simulink model "Scenario_TJunction_TrafficLights"  (R2021a)
settings: Solver=VariableStepAuto  StartTime=0.0  StopTime=15  RelTol=1e-3
model workspace (MAT data in the model file):
  Kz_dif = Simulink.Parameter
  Kz_dif.Value = Simulink.data.Expression
  Kz_dif.Value.ExpressionString = " L_dif / (Lc + ds)"
  Kz_dif.DataType = 'auto'
  Kz_dif.Dimensions = -1
  Kz_il = Simulink.Parameter
  Kz_il.Value = Simulink.data.Expression
  Kz_il.Value.ExpressionString = " L_il / (Lc + ds)"
  Kz_il.DataType = 'auto'
  Kz_il.Dimensions = -1
  Kz_ir = Simulink.Parameter
  Kz_ir.Value = Simulink.data.Expression
  Kz_ir.Value.ExpressionString = " L_ir / (Lc + ds)"
  Kz_ir.DataType = 'auto'
  Kz_ir.Dimensions = -1
  Kz_is = Simulink.Parameter
  Kz_is.Value = Simulink.data.Expression
  Kz_is.Value.ExpressionString = " L_is / (Lc + ds)"
  Kz_is.DataType = 'auto'
  Kz_is.Dimensions = -1
  Kz_long = Simulink.Parameter
  Kz_long.Value = Simulink.data.Expression
  Kz_long.Value.ExpressionString = " L_long / (Lc + ds)"
  Kz_long.Description = 'Segmentkapazität (wie viele autos passen hinein)'
  Kz_long.DataType = 'auto'
  Kz_long.Dimensions = -1
  Kz_pre = Simulink.Parameter
  Kz_pre.Value = Simulink.data.Expression
  Kz_pre.Value.ExpressionString = " L_pre / (Lc + ds)"
  Kz_pre.DataType = 'auto'
  Kz_pre.Dimensions = -1
  L_dif = Simulink.Parameter
  L_dif.Value = Simulink.data.Expression
  L_dif.Value.ExpressionString = "L_long-L_pre"
  L_dif.Description = 'Differenz zwischen Abbiegerspurlänge und normaler straßenlänge'
  L_dif.DataType = 'auto'
  L_dif.Dimensions = -1
  L_il = Simulink.Parameter
  L_il.Value = 30
  L_il.Description = 'Länge der innenkreuzungssegments, das linksabbieger durchqueren'
  L_il.DataType = 'auto'
  L_il.Dimensions = [1 1]
  L_ir = Simulink.Parameter
  L_ir.Value = 23
  L_ir.Description = 'Länge der innenkreuzungssegments, das rechtsabbieger durchqueren'
  L_ir.DataType = 'auto'
  L_ir.Dimensions = [1 1]
  L_is = Simulink.Parameter
  L_is.Value = 35
  L_is.Description = 'Länge der innenkreuzungssegments, das geradeausfahrer durchqueren'
  L_is.DataType = 'auto'
  L_is.Dimensions = [1 1]
  L_long = Simulink.Parameter
  L_long.Value = 52.8
  L_long.Description = 'Langes straßensegment  (52.8 meter)'
  L_long.DataType = 'auto'
  L_long.Dimensions = [1 1]
  L_pre = Simulink.Parameter
  L_pre.Value = 20
  L_pre.Description = 'Länge der Abbiegespuren'
  L_pre.DataType = 'auto'
  L_pre.Dimensions = [1 1]
  Lc = Simulink.Parameter
  Lc.Value = 4.4
  Lc.Description = 'Länge eines autos'
  Lc.DataType = 'auto'
  Lc.Dimensions = [1 1]
  Rk = Simulink.Parameter
  Rk.Value = Simulink.data.Expression
  Rk.Value.ExpressionString = " 1 / (Lc / v)"
  Rk.Description = 'Flussrate zwischen den Kanten (bei speed v)'
  Rk.DataType = 'auto'
  Rk.Dimensions = -1
  Tz_dif = Simulink.Parameter
  Tz_dif.Value = Simulink.data.Expression
  Tz_dif.Value.ExpressionString = " L_dif / v"
  Tz_dif.DataType = 'auto'
  Tz_dif.Dimensions = -1
  Tz_il = Simulink.Parameter
  Tz_il.Value = Simulink.data.Expression
  Tz_il.Value.ExpressionString = " L_il / v"
  Tz_il.DataType = 'auto'
  Tz_il.Dimensions = -1
  Tz_ir = Simulink.Parameter
  Tz_ir.Value = Simulink.data.Expression
  Tz_ir.Value.ExpressionString = " L_ir / v"
  Tz_ir.DataType = 'auto'
  Tz_ir.Dimensions = -1
  Tz_is = Simulink.Parameter
  Tz_is.Value = Simulink.data.Expression
  Tz_is.Value.ExpressionString = " L_is / v"
  Tz_is.DataType = 'auto'
  Tz_is.Dimensions = -1
  Tz_long = Simulink.Parameter
  Tz_long.Value = Simulink.data.Expression
  Tz_long.Value.ExpressionString = " L_long / v"
  Tz_long.Description = 'Segment durchfahrtzeit: wie lange würde ein auto brauchen,um
    | ungehindert durch das segment zu fahren.'
  Tz_long.DataType = 'auto'
  Tz_long.Dimensions = -1
  Tz_pre = Simulink.Parameter
  Tz_pre.Value = Simulink.data.Expression
  Tz_pre.Value.ExpressionString = " L_pre / v"
  Tz_pre.DataType = 'auto'
  Tz_pre.Dimensions = -1
  ds = Simulink.Parameter
  ds.Value = Simulink.data.Expression
  ds.Value.ExpressionString = "v*dt"
  ds.DataType = 'auto'
  ds.Dimensions = -1
  dt = Simulink.Parameter
  dt.Value = 1
  dt.Description = 'temporaler sicherheitsabstand'
  dt.DataType = 'auto'
  dt.Dimensions = [1 1]
  v = Simulink.Parameter
  v.Value = 13.89
  v.Description = 'geschwindigkeit eines autos
    | (km/h : 3.75 = m/s)
    | 	30km/h = 8,34m/s
    | 	20km/h = 5.56m/s
    | 	50km/h = 13.89m/s
    | '
  v.DataType = 'auto'
  v.Dimensions = [1 1]
libraries: StreetLanesLibrary x36, EdgesLibrary x36, SourcesAndSinksLibrary x12, LightsLibrary x2
settings Model: OrderedModelArguments=off  Creator=phill  LastModifiedBy=mariekutscher
settings SolverCC: ZeroCrossAlgorithm=Adaptive

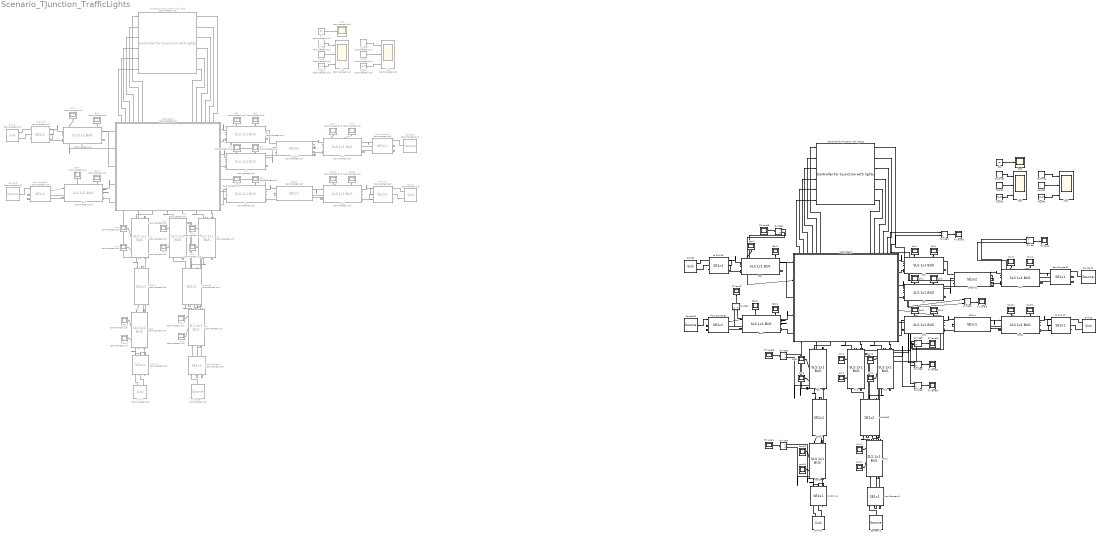
== system Scenario_TJunction_TrafficLights ==
  Ain : StreetLanesLibrary/SLS 1x1 BUS  Commented=on  Kz=Kz_dif  Tz=Tz_dif
  Ain1 : StreetLanesLibrary/SLS 1x1 BUS  Kz=Kz_dif  Tz=Tz_dif
  AinSplit1 : EdgesLibrary/SE1x2  Commented=on  Rk1=0.5*Rk  Rk2=0.5*Rk
  AinSplit2 : EdgesLibrary/SE1x2  Rk1=0.5*Rk  Rk2=0.5*Rk
  AinX : Scope  Commented=on
  AinX1 : Scope
  AinY : Scope  Commented=on
  AinY1 : Scope
  Ali : StreetLanesLibrary/SLS 1x1 BUS  Commented=on  Kz=Kz_pre  Tz=Tz_pre
  Ali1 : StreetLanesLibrary/SLS 1x1 BUS  Kz=Kz_pre  Tz=Tz_pre
  AliX : Scope  Commented=on
  AliX1 : Scope
  AliY : Scope  Commented=on
  AliY1 : Scope
  Ao : StreetLanesLibrary/SLS 1x1 BUS  Commented=on  Kz=Kz_pre  Tz=Tz_pre
  Ao1 : StreetLanesLibrary/SLS 1x1 BUS  Kz=Kz_pre  Tz=Tz_pre
  AoX : Scope  Commented=on
  AoX1 : Scope
  AoY : Scope  Commented=on
  AoY1 : Scope
  Aout : StreetLanesLibrary/SLS 1x1 BUS  Commented=on  Kz=Kz_dif  Tz=Tz_dif
  Aout1 : StreetLanesLibrary/SLS 1x1 BUS  Kz=Kz_dif  Tz=Tz_dif
  AoutX : Scope  Commented=on
  AoutX1 : Scope
  AoutY : Scope  Commented=on
  AoutY1 : Scope
  Ari : StreetLanesLibrary/SLS 1x1 BUS  Commented=on  Kz=Kz_pre  Tz=Tz_pre
  Ari1 : StreetLanesLibrary/SLS 1x1 BUS  Kz=Kz_pre  Tz=Tz_pre
  AriX : Scope  Commented=on
  AriX1 : Scope
  AriY : Scope  Commented=on
  AriY1 : Scope
  Bo : StreetLanesLibrary/SLS 1x1 BUS  Commented=on  Kz=Kz_pre  Tz=Tz_pre
  Bo1 : StreetLanesLibrary/SLS 1x1 BUS  Kz=Kz_pre  Tz=Tz_pre
  BoX : Scope  Commented=on
  BoX1 : Scope
  BoY : Scope  Commented=on
  BoY1 : Scope
  Brs : StreetLanesLibrary/SLS 1x1 BUS  Commented=on  Kz=Kz_pre  Tz=Tz_pre
  Brs1 : StreetLanesLibrary/SLS 1x1 BUS  Kz=Kz_pre  Tz=Tz_pre
  BrsX : Scope  Commented=on
  BrsX1 : Scope
  BrsY : Scope  Commented=on
  BrsY1 : Scope
  Cin : StreetLanesLibrary/SLS 1x1 BUS  Commented=on  Kz=Kz_dif  Tz=Tz_dif
  Cin1 : StreetLanesLibrary/SLS 1x1 BUS  Kz=Kz_dif  Tz=Tz_dif
  CinSplit : EdgesLibrary/SE1x2  Commented=on  Rk1=0.5*Rk  Rk2=0.5*Rk
  CinSplit1 : EdgesLibrary/SE1x2  Rk1=0.5*Rk  Rk2=0.5*Rk
  CinX : Scope  Commented=on
  CinX1 : Scope
  CinY : Scope  Commented=on
  CinY1 : Scope
  Cl : StreetLanesLibrary/SLS 1x1 BUS  Commented=on  Kz=Kz_pre  Tz=Tz_pre
  Cl1 : StreetLanesLibrary/SLS 1x1 BUS  Kz=Kz_pre  Tz=Tz_pre
  ClX : Scope  Commented=on
  ClX1 : Scope
  ClY : Scope  Commented=on
  ClY1 : Scope
  Co : StreetLanesLibrary/SLS 1x1 BUS  Commented=on  Kz=Kz_pre  Tz=Tz_pre
  Co1 : StreetLanesLibrary/SLS 1x1 BUS  Kz=Kz_pre  Tz=Tz_pre
  CoX : Scope  Commented=on
  CoX1 : Scope
  CoY : Scope  Commented=on
  CoY1 : Scope
  Controller for t-junction with lights : LightsLibrary/Controller for t-junction with lights  Commented=on  green_time=10
  Controller for t-junction with lights1 : LightsLibrary/Controller for t-junction with lights  green_time=10
  Cout : StreetLanesLibrary/SLS 1x1 BUS  Commented=on  Kz=Kz_dif  Tz=Tz_dif
  Cout1 : StreetLanesLibrary/SLS 1x1 BUS  Kz=Kz_dif  Tz=Tz_dif
  CoutX : Scope  Commented=on
  CoutX1 : Scope
  CoutY : Scope  Commented=on
  CoutY1 : Scope
  Cs : StreetLanesLibrary/SLS 1x1 BUS  Commented=on  Kz=Kz_pre  Tz=Tz_pre
  Cs1 : StreetLanesLibrary/SLS 1x1 BUS  Kz=Kz_pre  Tz=Tz_pre
  CsX : Scope  Commented=on
  CsX1 : Scope
  CsY : Scope  Commented=on
  CsY1 : Scope
  Divide{,1..9} (10 alike) : Product  Inputs=*/
  Kz_dif : Constant  Commented=on  Value=Kz_dif
  Kz_dif1 : Constant  Value=Kz_dif
  Kz_long : Constant  Commented=on  Value=Kz_long
  Kz_long1 : Constant  Value=Kz_long
  Kz_pre : Constant  Commented=on  Value=Kz_pre
  Kz_pre1 : Constant  Value=Kz_pre
  Kzs : Scope  Commented=on  NumInputPorts=3
  Kzs1 : Scope  NumInputPorts=3
  Rk : Constant  Commented=on  Value=Rk
  Rk1 : Constant  Value=Rk
  SE1x1 : EdgesLibrary/SE1x1  Commented=on  Rk=Rk
  SE1x2 : EdgesLibrary/SE1x1  Rk=Rk
  SE1x3 : EdgesLibrary/SE1x1  Commented=on  Rk=Rk
  SE1x4 : EdgesLibrary/SE1x1  Rk=Rk
  Sink A : SourcesAndSinksLibrary/Sink  Commented=on  SystemSampleTime=-1  VariantActivationTime=update diagram  Latency=0  AutoFrameSizeCalculation=off
      settings: PortSchema="{\"entries\":[{\"content\":{\"sides\":[{\"content\":{\"connectorIds\":[\"Out1\",\"Out2\"]},\"type\":\"ConnectorPlacement.EquallySpacedRectSide\",\"uuid\":\"9fd2383e-3590-4f0f-bafc-5a4adfbb32b4\"},{\"content\":{\"connectorIds\":[],\"side\":\"RIGHT\"},\"type\":\"ConnectorPlacement.EquallySpacedRectSide\",\"uuid\":\"1e687aa9-1098-45bd-a1f6-ea403f3f2897\"},{\"content\":{\"connectorIds\":[],\"side\":\"TOP\"},\"type\":\"ConnectorPlacement.EquallySpacedRectSide\",\"uuid\":\"fe6eaa71-085c-414b-983a-a0e72e52a49c\"}]},\"type\":\"ConnectorPlacement.EquallySpacedConnector\",\"uuid\":\"370c1712-4373-4726-99c2-6cb04807ece1\"}],\"packageUris\":[\"http://schema.mathworks.com/mf0/Connector/R2020b\"],\"version\":\"1.0\"}"
  Sink A1 : SourcesAndSinksLibrary/Sink  SystemSampleTime=-1  VariantActivationTime=update diagram  Latency=0  AutoFrameSizeCalculation=off
      settings: PortSchema="{\"entries\":[{\"content\":{\"sides\":[{\"content\":{\"connectorIds\":[\"Out1\",\"Out2\"]},\"type\":\"ConnectorPlacement.EquallySpacedRectSide\",\"uuid\":\"9fd2383e-3590-4f0f-bafc-5a4adfbb32b4\"},{\"content\":{\"connectorIds\":[],\"side\":\"RIGHT\"},\"type\":\"ConnectorPlacement.EquallySpacedRectSide\",\"uuid\":\"1e687aa9-1098-45bd-a1f6-ea403f3f2897\"},{\"content\":{\"connectorIds\":[],\"side\":\"TOP\"},\"type\":\"ConnectorPlacement.EquallySpacedRectSide\",\"uuid\":\"fe6eaa71-085c-414b-983a-a0e72e52a49c\"}]},\"type\":\"ConnectorPlacement.EquallySpacedConnector\",\"uuid\":\"370c1712-4373-4726-99c2-6cb04807ece1\"}],\"packageUris\":[\"http://schema.mathworks.com/mf0/Connector/R2020b\"],\"version\":\"1.0\"}"
  Sink B : SourcesAndSinksLibrary/Sink  Commented=on  SystemSampleTime=-1  VariantActivationTime=update diagram  Latency=0  AutoFrameSizeCalculation=off
      settings: PortSchema="{\"entries\":[{\"content\":{\"sides\":[{\"content\":{\"connectorIds\":[\"Out1\",\"Out2\"]},\"type\":\"ConnectorPlacement.EquallySpacedRectSide\",\"uuid\":\"9fd2383e-3590-4f0f-bafc-5a4adfbb32b4\"},{\"content\":{\"connectorIds\":[],\"side\":\"RIGHT\"},\"type\":\"ConnectorPlacement.EquallySpacedRectSide\",\"uuid\":\"1e687aa9-1098-45bd-a1f6-ea403f3f2897\"},{\"content\":{\"connectorIds\":[],\"side\":\"TOP\"},\"type\":\"ConnectorPlacement.EquallySpacedRectSide\",\"uuid\":\"fe6eaa71-085c-414b-983a-a0e72e52a49c\"}]},\"type\":\"ConnectorPlacement.EquallySpacedConnector\",\"uuid\":\"370c1712-4373-4726-99c2-6cb04807ece1\"}],\"packageUris\":[\"http://schema.mathworks.com/mf0/Connector/R2020b\"],\"version\":\"1.0\"}"
  Sink B1 : SourcesAndSinksLibrary/Sink  SystemSampleTime=-1  VariantActivationTime=update diagram  Latency=0  AutoFrameSizeCalculation=off
      settings: PortSchema="{\"entries\":[{\"content\":{\"sides\":[{\"content\":{\"connectorIds\":[\"Out1\",\"Out2\"]},\"type\":\"ConnectorPlacement.EquallySpacedRectSide\",\"uuid\":\"9fd2383e-3590-4f0f-bafc-5a4adfbb32b4\"},{\"content\":{\"connectorIds\":[],\"side\":\"RIGHT\"},\"type\":\"ConnectorPlacement.EquallySpacedRectSide\",\"uuid\":\"1e687aa9-1098-45bd-a1f6-ea403f3f2897\"},{\"content\":{\"connectorIds\":[],\"side\":\"TOP\"},\"type\":\"ConnectorPlacement.EquallySpacedRectSide\",\"uuid\":\"fe6eaa71-085c-414b-983a-a0e72e52a49c\"}]},\"type\":\"ConnectorPlacement.EquallySpacedConnector\",\"uuid\":\"370c1712-4373-4726-99c2-6cb04807ece1\"}],\"packageUris\":[\"http://schema.mathworks.com/mf0/Connector/R2020b\"],\"version\":\"1.0\"}"
  Sink C : SourcesAndSinksLibrary/Sink  Commented=on  SystemSampleTime=-1  VariantActivationTime=update diagram  Latency=0  AutoFrameSizeCalculation=off
      settings: PortSchema="{\"entries\":[{\"content\":{\"sides\":[{\"content\":{\"connectorIds\":[\"Out1\",\"Out2\"]},\"type\":\"ConnectorPlacement.EquallySpacedRectSide\",\"uuid\":\"9fd2383e-3590-4f0f-bafc-5a4adfbb32b4\"},{\"content\":{\"connectorIds\":[],\"side\":\"RIGHT\"},\"type\":\"ConnectorPlacement.EquallySpacedRectSide\",\"uuid\":\"1e687aa9-1098-45bd-a1f6-ea403f3f2897\"},{\"content\":{\"connectorIds\":[],\"side\":\"TOP\"},\"type\":\"ConnectorPlacement.EquallySpacedRectSide\",\"uuid\":\"fe6eaa71-085c-414b-983a-a0e72e52a49c\"}]},\"type\":\"ConnectorPlacement.EquallySpacedConnector\",\"uuid\":\"370c1712-4373-4726-99c2-6cb04807ece1\"}],\"packageUris\":[\"http://schema.mathworks.com/mf0/Connector/R2020b\"],\"version\":\"1.0\"}"
  Sink C1 : SourcesAndSinksLibrary/Sink  SystemSampleTime=-1  VariantActivationTime=update diagram  Latency=0  AutoFrameSizeCalculation=off
      settings: PortSchema="{\"entries\":[{\"content\":{\"sides\":[{\"content\":{\"connectorIds\":[\"Out1\",\"Out2\"]},\"type\":\"ConnectorPlacement.EquallySpacedRectSide\",\"uuid\":\"9fd2383e-3590-4f0f-bafc-5a4adfbb32b4\"},{\"content\":{\"connectorIds\":[],\"side\":\"RIGHT\"},\"type\":\"ConnectorPlacement.EquallySpacedRectSide\",\"uuid\":\"1e687aa9-1098-45bd-a1f6-ea403f3f2897\"},{\"content\":{\"connectorIds\":[],\"side\":\"TOP\"},\"type\":\"ConnectorPlacement.EquallySpacedRectSide\",\"uuid\":\"fe6eaa71-085c-414b-983a-a0e72e52a49c\"}]},\"type\":\"ConnectorPlacement.EquallySpacedConnector\",\"uuid\":\"370c1712-4373-4726-99c2-6cb04807ece1\"}],\"packageUris\":[\"http://schema.mathworks.com/mf0/Connector/R2020b\"],\"version\":\"1.0\"}"
  Source A : SourcesAndSinksLibrary/Source  Commented=on  SystemSampleTime=-1  VariantActivationTime=update diagram  Latency=0  AutoFrameSizeCalculation=off
  Source A1 : SourcesAndSinksLibrary/Source  SystemSampleTime=-1  VariantActivationTime=update diagram  Latency=0  AutoFrameSizeCalculation=off
  Source B : SourcesAndSinksLibrary/Source  Commented=on  SystemSampleTime=-1  VariantActivationTime=update diagram  Latency=0  AutoFrameSizeCalculation=off
  Source B1 : SourcesAndSinksLibrary/Source  SystemSampleTime=-1  VariantActivationTime=update diagram  Latency=0  AutoFrameSizeCalculation=off
  Source C : SourcesAndSinksLibrary/Source  Commented=on  SystemSampleTime=-1  VariantActivationTime=update diagram  Latency=0  AutoFrameSizeCalculation=off
  Source C1 : SourcesAndSinksLibrary/Source  SystemSampleTime=-1  VariantActivationTime=update diagram  Latency=0  AutoFrameSizeCalculation=off
  Subsystem1 : Subsystem  Commented=on  mask{Kz_left=Kz_il, Tz_left=Tz_il, Kz_straight=Kz_is, Tz_straight=Tz_is, Kz_right=Kz_ir, Tz_right=Tz_ir, Rk=Rk}
      settings: PortSchema="{\"entries\":[{\"content\":{\"sides\":[{\"content\":{\"connectorIds\":[\"In1\",\"In2\",\"Out24\",\"In3\",\"Out25\"]},\"type\":\"ConnectorPlacement.EquallySpacedRectSide\",\"uuid\":\"96c9f498-b0bc-4839-a476-8992d885d35a\"},{\"content\":{\"connectorIds\":[\"In14\",\"Out1\",\"In15\",\"Out2\",\"In16\",\"In17\",\"Out3\"],\"side\":\"RIGHT\"},\"type\":\"ConnectorPlacement.EquallySpacedRectSide\",\"uuid\":\"11ab0cdd-7db6-4f39-a252-8216aa6322d2\"},{\"content\":{\"connectorIds\":[\"Out7\",\"Out8\",\"Out9\",\"Out10\",\"Out11\",\"Out12\",\"Out13\",\"Out14\",\"Out15\",\"Out16\",\"Out17\",\"Out18\",\"Out19\",\"Out20\",\"Out21\",\"Out22\",\"Out23\",\"In4\",\"In5\",\"In6\",\"In7\",\"In8\",\"In9\"],\"side\":\"TOP\"},\"type\":\"ConnectorPlacement.EquallySpacedRectSide\",\"uuid\":\"f8ff7b80-df82-4633-b83a-80e44c4409b9\"},{\"content\":{\"connectorIds\":[\"In10\",\"In11\",\"Out4\",\"In12\",\"Out5\",\"In13\",\"Out6\"],\"side\":\"BOTTOM\"},\"type\":\"ConnectorPlacement.EquallySpacedRectSide\",\"uuid\":\"816219a6-152c-447e-807e-ad4d62c96b47\"}]},\"type\":\"ConnectorPlacement.EquallySpacedConnector\",\"uuid\":\"16c591aa-9a6b-4cb9-9c60-a78ca06e8a6b\"}],\"packageUris\":[\"http://schema.mathworks.com/mf0/Connector/R2020b\"],\"version\":\"1.0\"}"
      mask Display:
      | %image('$imagefile'); % Use "Edit Image" on toolstrip to change.
      | disp('T \n\n');
      | KzS = get_param(gcb,'Kz_straight');
      | TzS = get_param(gcb,'Tz_straight');
      | KzR = get_param(gcb,'Kz_right');
      | TzR = get_param(gcb,'Tz_right');
      | KzL = get_param(gcb,'Kz_left');
      | TzL = get_param(gcb,'Tz_left');
      | Rk = get_param(gcb,'Rk');
      | disp(['Rk = ', Rk, ' | Kz/Tz L = ', KzL, ' ', TzL, ' | Kz/Tz S = ', KzS, ' ', TzS, ' | Kz/Tz R = ', KzR, ' ', TzR]);
  Subsystem2 : Subsystem  mask{Kz_left=Kz_il, Tz_left=Tz_il, Kz_straight=Kz_is, Tz_straight=Tz_is, Kz_right=Kz_ir, Tz_right=Tz_ir, Rk=Rk}
      settings: PortSchema="{\"entries\":[{\"content\":{\"sides\":[{\"content\":{\"connectorIds\":[\"In1\",\"In2\",\"Out24\",\"In3\",\"Out25\"]},\"type\":\"ConnectorPlacement.EquallySpacedRectSide\",\"uuid\":\"96c9f498-b0bc-4839-a476-8992d885d35a\"},{\"content\":{\"connectorIds\":[\"In14\",\"Out1\",\"In15\",\"Out2\",\"In16\",\"In17\",\"Out3\"],\"side\":\"RIGHT\"},\"type\":\"ConnectorPlacement.EquallySpacedRectSide\",\"uuid\":\"11ab0cdd-7db6-4f39-a252-8216aa6322d2\"},{\"content\":{\"connectorIds\":[\"Out7\",\"Out8\",\"Out9\",\"Out10\",\"Out11\",\"Out12\",\"Out13\",\"Out14\",\"Out15\",\"Out16\",\"Out17\",\"Out18\",\"Out19\",\"Out20\",\"Out21\",\"Out22\",\"Out23\",\"In4\",\"In5\",\"In6\",\"In7\",\"In8\",\"In9\"],\"side\":\"TOP\"},\"type\":\"ConnectorPlacement.EquallySpacedRectSide\",\"uuid\":\"f8ff7b80-df82-4633-b83a-80e44c4409b9\"},{\"content\":{\"connectorIds\":[\"In10\",\"In11\",\"Out4\",\"In12\",\"Out5\",\"In13\",\"Out6\"],\"side\":\"BOTTOM\"},\"type\":\"ConnectorPlacement.EquallySpacedRectSide\",\"uuid\":\"816219a6-152c-447e-807e-ad4d62c96b47\"}]},\"type\":\"ConnectorPlacement.EquallySpacedConnector\",\"uuid\":\"16c591aa-9a6b-4cb9-9c60-a78ca06e8a6b\"}],\"packageUris\":[\"http://schema.mathworks.com/mf0/Connector/R2020b\"],\"version\":\"1.0\"}"
      mask Display:
      | %image('$imagefile'); % Use "Edit Image" on toolstrip to change.
      | disp('T \n\n');
      | KzS = get_param(gcb,'Kz_straight');
      | TzS = get_param(gcb,'Tz_straight');
      | KzR = get_param(gcb,'Kz_right');
      | TzR = get_param(gcb,'Tz_right');
      | KzL = get_param(gcb,'Kz_left');
      | TzL = get_param(gcb,'Tz_left');
      | Rk = get_param(gcb,'Rk');
      | disp(['Rk = ', Rk, ' | Kz/Tz L = ', KzL, ' ', TzL, ' | Kz/Tz S = ', KzS, ' ', TzS, ' | Kz/Tz R = ', KzR, ' ', TzR]);
  Tz_dif : Constant  Commented=on  Value=Tz_dif
  Tz_dif1 : Constant  Value=Tz_dif
  Tz_long : Constant  Commented=on  Value=Tz_long
  Tz_long1 : Constant  Value=Tz_long
  Tz_pre : Constant  Commented=on  Value=Tz_pre
  Tz_pre1 : Constant  Value=Tz_pre
  Tzs : Scope  Commented=on  NumInputPorts=3
  Tzs1 : Scope  Commented=on
  Tzs2 : Scope  NumInputPorts=3
  Tzs3 : Scope
  fill level{,1..9} (10 alike) : Scope
  from Source A : EdgesLibrary/SE1x1  Commented=on  Rk=Rk
  from Source A1 : EdgesLibrary/SE1x1  Rk=Rk
  from Source B : EdgesLibrary/SE1x1  Commented=on  Rk=Rk
  from Source B1 : EdgesLibrary/SE1x1  Rk=Rk
  from Source C : EdgesLibrary/SE1x1  Commented=on  Rk=Rk
  from Source C1 : EdgesLibrary/SE1x1  Rk=Rk
  to Sink A : EdgesLibrary/SE1x1  Commented=on  Rk=Rk
  to Sink A1 : EdgesLibrary/SE1x1  Rk=Rk
  to Sink B : EdgesLibrary/SE1x1  Commented=on  Rk=Rk
  to Sink B1 : EdgesLibrary/SE1x1  Rk=Rk
  to Sink C : EdgesLibrary/SE1x1  Commented=on  Rk=Rk
  to Sink C1 : EdgesLibrary/SE1x1  Rk=Rk
  wires:
  Ao/6 -> Subsystem1/10(Ao x)
  Ao/7 -> Subsystem1/11(Ao Kz)
  Subsystem1/4(Ao yk) -> Ao/1
  Ali/2 -> Subsystem1/12(Ali x0)
  Subsystem1/5(Ali yk) -> Ali/2
  Ari/2 -> Subsystem1/13(Ari x0)
  Subsystem1/6(Ari yk) -> Ari/2
  Ari/7 -> AinSplit1/5
  Ari/6 -> AinSplit1/4
  Ali/7 -> AinSplit1/3
  Ali/6 -> AinSplit1/2
  Ao/2 -> SE1x1/1
  SE1x1/2 -> Ao/2
  Ain/2 -> AinSplit1/1
  Aout/6 -> SE1x1/2
  Aout/7 -> SE1x1/3
  SE1x1/1 -> Aout/1
  Source A/1 -> from Source A/1
  from Source A/1 -> Ain/1
  Ain/7 -> from Source A/3
  Ain/6 -> from Source A/2
  to Sink A/2 -> Aout/2
  Aout/2 -> to Sink A/1
  Sink A/1 -> to Sink A/2
  Sink A/2 -> to Sink A/3
  Co/6 -> Subsystem1/16(Co x)
  Co/7 -> Subsystem1/17(Co Kz)
  Subsystem1/3(Co yk) -> Co/1
  Subsystem1/2(Cl yk) -> Cl/2
  Cl/2 -> Subsystem1/15(Cl x0)
  Subsystem1/1(Cs yk) -> Cs/2
  Cs/2 -> Subsystem1/14(Cs x0)
  Bo/6 -> Subsystem1/1(Bo x)
  Bo/7 -> Subsystem1/2(Bo Kz)
  Subsystem1/24(Bo yk) -> Bo/1
  Brs/2 -> Subsystem1/3(Brs x0)
  Subsystem1/25(Brs yk) -> Brs/2
  SE1x3/2 -> Co/2
  Co/2 -> SE1x3/1
  SE1x3/1 -> Cout/1
  Cout/7 -> SE1x3/3
  Cout/6 -> SE1x3/2
  Cs/6 -> CinSplit/2
  Cs/7 -> CinSplit/3
  CinSplit/1 -> Cs/1
  Cl/6 -> CinSplit/4
  Cl/7 -> CinSplit/5
  CinSplit/2 -> Cl/1
  CinSplit/3 -> Cin/2
  Cin/2 -> CinSplit/1
  Sink C/1 -> to Sink C/2
  Sink C/2 -> to Sink C/3
  Cout/2 -> to Sink C/1
  to Sink C/2 -> Cout/2
  Source C/1 -> from Source C/1
  Cin/6 -> from Source C/2
  Cin/7 -> from Source C/3
  from Source C/1 -> Cin/1
  Source B/1 -> from Source B/1
  Sink B/2 -> to Sink B/3
  Sink B/1 -> to Sink B/2
  Bo/2 -> to Sink B/1
  to Sink B/2 -> Bo/2
  Brs/6 -> from Source B/2
  Brs/7 -> from Source B/3
  from Source B/1 -> Brs/1
  Bo/4 -> BoY/1
  Cs/4 -> CsY/1
  Cl/4 -> ClY/1
  Cl/3 -> ClX/1
  Co/3 -> CoX/1
  Co/4 -> CoY/1
  Cs/3 -> CsX/1
  Brs/3 -> BrsX/1
  Brs/4 -> BrsY/1
  Bo/3 -> BoX/1
  Cin/4 -> CinY/1
  Cin/3 -> CinX/1
  Cout/3 -> CoutX/1
  Cout/4 -> CoutY/1
  Ao/3 -> AoX/1
  Ao/4 -> AoY/1
  Ali/4 -> AliY/1
  Ali/3 -> AliX/1
  Ari/4 -> AriY/1
  Ari/3 -> AriX/1
  Aout/3 -> AoutX/1
  Aout/4 -> AoutY/1
  Ain/4 -> AinY/1
  Ain/3 -> AinX/1
  Tz_long/1 -> Tzs/1  "Tz_long"
  Tz_pre/1 -> Tzs/2  "Tz_pre"
  Tz_dif/1 -> Tzs/3  "Tz_dif"
  Kz_long/1 -> Kzs/1  "Kz_long"
  Kz_pre/1 -> Kzs/2  "Kz_pre"
  Kz_dif/1 -> Kzs/3  "Kz_dif"
  Rk/1 -> Tzs1/1  "Rk"
  AinSplit1/3 -> Ain/2
  AinSplit1/2 -> Ari/1
  AinSplit1/1 -> Ali/1
  Subsystem1/12(free_1) -> Controller for t-junction with lights/1
  Subsystem1/11(free_2) -> Controller for t-junction with lights/2
  Subsystem1/9(free_4) -> Controller for t-junction with lights/4
  Subsystem1/8(free_5) -> Controller for t-junction with lights/5
  Subsystem1/7(free_6) -> Controller for t-junction with lights/6
  Subsystem1/10(free_3) -> Controller for t-junction with lights/3
  Controller for t-junction with lights/1 -> Subsystem1/9(Cs8)
  Controller for t-junction with lights/2 -> Subsystem1/8(Cl7)
  Controller for t-junction with lights/3 -> Subsystem1/7(Ari4)
  Controller for t-junction with lights/4 -> Subsystem1/6(Ali3)
  Controller for t-junction with lights/5 -> Subsystem1/5(Brs12)
  Controller for t-junction with lights/6 -> Subsystem1/4(Brs11)
  Bo1/7 -> Divide8/2, Subsystem2/2(Bo Kz)
  AinSplit2/1 -> Ali1/1
  Sink C1/2 -> to Sink C1/3
  Cin1/6 -> Divide/1, from Source C1/2
  to Sink A1/2 -> Aout1/2
  Subsystem2/3(Co yk) -> Co1/1
  Cl1/4 -> ClY1/1
  from Source C1/1 -> Cin1/1
  from Source B1/1 -> Brs1/1
  from Source A1/1 -> Ain1/1
  Brs1/3 -> BrsX1/1
  Kz_pre1/1 -> Kzs1/2  "Kz_pre"
  Co1/2 -> SE1x4/1
  Ari1/2 -> Subsystem2/13(Ari x0)
  Cs1/3 -> CsX1/1
  Controller for t-junction with lights1/2 -> Subsystem2/8(Cl7)
  Cl1/7 -> Divide2/2, CinSplit1/5
  Cin1/7 -> Divide/2, from Source C1/3
  Sink A1/1 -> to Sink A1/2
  Cout1/2 -> to Sink C1/1
  Ari1/7 -> Divide5/2, AinSplit2/5
  AinSplit2/3 -> Ain1/2
  Source B1/1 -> from Source B1/1
  Cout1/4 -> CoutY1/1
  Co1/7 -> Subsystem2/17(Co Kz), Divide9/2
  Subsystem2/2(Cl yk) -> Cl1/2
  CinSplit1/3 -> Cin1/2
  Sink C1/1 -> to Sink C1/2
  Ali1/2 -> Subsystem2/12(Ali x0)
  Subsystem2/6(Ari yk) -> Ari1/2
  Ali1/7 -> Divide6/2, AinSplit2/3
  Brs1/7 -> Divide7/2, from Source B1/3
  Cs1/4 -> CsY1/1
  Source C1/1 -> from Source C1/1
  Ain1/3 -> AinX1/1
  Rk1/1 -> Tzs3/1  "Rk"
  Controller for t-junction with lights1/4 -> Subsystem2/6(Ali3)
  SE1x4/1 -> Cout1/1
  Aout1/3 -> AoutX1/1
  Aout1/4 -> AoutY1/1
  Co1/6 -> Divide9/1, Subsystem2/16(Co x)
  Subsystem2/8(free_5) -> Controller for t-junction with lights1/5
  SE1x2/1 -> Aout1/1
  Ari1/3 -> AriX1/1
  Bo1/2 -> to Sink B1/1
  Brs1/6 -> from Source B1/2, Divide7/1
  Cout1/7 -> SE1x4/3
  Ain1/7 -> from Source A1/3
  Tz_pre1/1 -> Tzs2/2  "Tz_pre"
  Cout1/3 -> CoutX1/1
  Sink A1/2 -> to Sink A1/3
  Sink B1/2 -> to Sink B1/3
  Subsystem2/4(Ao yk) -> Ao1/1
  Co1/3 -> CoX1/1
  Sink B1/1 -> to Sink B1/2
  Cl1/2 -> Subsystem2/15(Cl x0)
  Ali1/6 -> AinSplit2/2, Divide6/1
  Subsystem2/1(Cs yk) -> Cs1/2
  Cs1/2 -> Subsystem2/14(Cs x0)
  Ari1/6 -> Divide5/1, AinSplit2/4
  Ari1/4 -> AriY1/1
  Cl1/6 -> Divide2/1, CinSplit1/4
  Bo1/4 -> BoY1/1
  Kz_long1/1 -> Kzs1/1  "Kz_long"
  Aout1/7 -> SE1x2/3, Divide4/2
  Kz_dif1/1 -> Kzs1/3  "Kz_dif"
  Bo1/6 -> Divide8/1, Subsystem2/1(Bo x)
  Subsystem2/7(free_6) -> Controller for t-junction with lights1/6
  Cl1/3 -> ClX1/1
  SE1x4/2 -> Co1/2
  Cs1/6 -> Divide1/1, CinSplit1/2
  Cout1/6 -> SE1x4/2
  CinSplit1/1 -> Cs1/1
  CinSplit1/2 -> Cl1/1
  Cs1/7 -> Divide1/2, CinSplit1/3
  Aout1/2 -> to Sink A1/1
  to Sink B1/2 -> Bo1/2
  Aout1/6 -> Divide4/1, SE1x2/2
  Cin1/4 -> CinY1/1
  Ao1/3 -> AoX1/1
  Subsystem2/25(Brs yk) -> Brs1/2
  AinSplit2/2 -> Ari1/1
  Ain1/6 -> from Source A1/2
  Ain1/4 -> AinY1/1
  to Sink C1/2 -> Cout1/2
  Controller for t-junction with lights1/6 -> Subsystem2/4(Brs11)
  Subsystem2/10(free_3) -> Controller for t-junction with lights1/3
  Brs1/2 -> Subsystem2/3(Brs x0)
  Brs1/4 -> BrsY1/1
  Co1/4 -> CoY1/1
  Controller for t-junction with lights1/3 -> Subsystem2/7(Ari4)
  Tz_dif1/1 -> Tzs2/3  "Tz_dif"
  Ali1/3 -> AliX1/1
  Source A1/1 -> from Source A1/1
  Subsystem2/11(free_2) -> Controller for t-junction with lights1/2
  Subsystem2/12(free_1) -> Controller for t-junction with lights1/1
  Cin1/2 -> CinSplit1/1
  Ao1/4 -> AoY1/1
  Subsystem2/9(free_4) -> Controller for t-junction with lights1/4
  Controller for t-junction with lights1/5 -> Subsystem2/5(Brs12)
  Bo1/3 -> BoX1/1
  Ali1/4 -> AliY1/1
  Tz_long1/1 -> Tzs2/1  "Tz_long"
  Controller for t-junction with lights1/1 -> Subsystem2/9(Cs8)
  Subsystem2/24(Bo yk) -> Bo1/1
  Cin1/3 -> CinX1/1
  Ao1/2 -> SE1x2/1
  SE1x2/2 -> Ao1/2
  Ain1/2 -> AinSplit2/1
  Subsystem2/5(Ali yk) -> Ali1/2
  Divide/1 -> fill level/1
  Divide1/1 -> fill level1/1
  Divide2/1 -> fill level2/1
  Divide3/1 -> fill level3/1
  Ao1/7 -> Divide3/2, Subsystem2/11(Ao Kz)
  Ao1/6 -> Divide3/1, Subsystem2/10(Ao x)
  Divide4/1 -> fill level4/1
  Divide5/1 -> fill level5/1
  Divide6/1 -> fill level6/1
  Divide7/1 -> fill level7/1
  Divide8/1 -> fill level8/1
  Divide9/1 -> fill level9/1

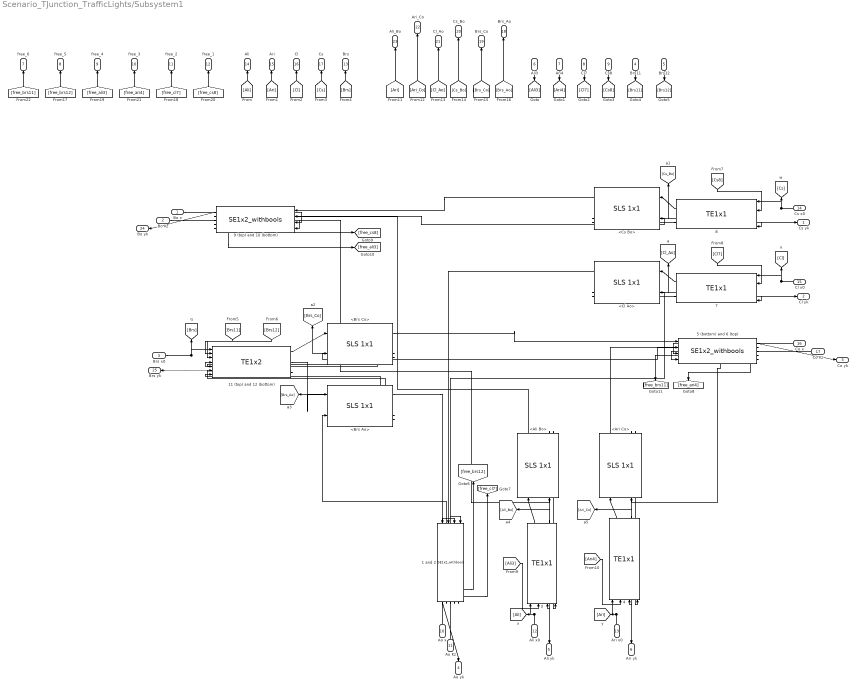
== system Scenario_TJunction_TrafficLights/Subsystem1 ==
  Bo x : Inport
  Bo Kz : Inport  Port=2
  Brs x0 : Inport  Port=3
  Brs11 : Inport  Port=4
  Brs12 : Inport  Port=5
  Ali3 : Inport  Port=6
  Ari4 : Inport  Port=7
  Cl7 : Inport  Port=8
  Cs8 : Inport  Port=9
  Ao x : Inport  Port=10
  Ao Kz : Inport  Port=11
  Ali x0 : Inport  Port=12
  Ari x0 : Inport  Port=13
  Cs x0 : Inport  Port=14
  Cl x0 : Inport  Port=15
  Co x : Inport  Port=16
  Co Kz : Inport  Port=17
  " 5 (bottom) and 6 (top)" : EdgesLibrary/SE1x2_withbools  Rk1=Rk  Rk2=Rk
  1 and 2 : EdgesLibrary/SE1x2_withbools  Rk1=Rk  Rk2=Rk
  11 (top) and 12 (bottom) : EdgesLibrary/TE1x2  Rk1=0.5*Rk  Rk2=0.5*Rk
  {3..4,7..8} (4 alike) : EdgesLibrary/TE1x1  Rk=Rk
  9 (top) and 10 (bottom) : EdgesLibrary/SE1x2_withbools  Rk1=Rk  Rk2=Rk
  <Ali Bo> : StreetLanesLibrary/SLS 1x1  Kz=Kz_left  Tz=Tz_left
  <Ari Co> : StreetLanesLibrary/SLS 1x1  Kz=Kz_right  Tz=Tz_right
  <Brs Ao> : StreetLanesLibrary/SLS 1x1  Kz=Kz_right  Tz=Tz_right
  <Brs Co> : StreetLanesLibrary/SLS 1x1  Kz=Kz_straight  Tz=Tz_straight
  <Cl Ao> : StreetLanesLibrary/SLS 1x1  Kz=Kz_left  Tz=Tz_left
  <Cs Bo> : StreetLanesLibrary/SLS 1x1  Kz=Kz_straight  Tz=Tz_straight
  Cs yk : Outport
  Cl yk : Outport  Port=2
  Co yk : Outport  Port=3
  Ao yk : Outport  Port=4
  Ali yk : Outport  Port=5
  Ari yk : Outport  Port=6
  free_6 : Outport  Port=7
  free_5 : Outport  Port=8
  free_4 : Outport  Port=9
  free_3 : Outport  Port=10
  free_2 : Outport  Port=11
  free_1 : Outport  Port=12
  Brs : Outport  Port=13
  Ali : Outport  Port=14
  Ari : Outport  Port=15
  Cl : Outport  Port=16
  Cs : Outport  Port=17
  Brs_Ao : Outport  Port=18
  Brs_Co : Outport  Port=19
  Cs_Bo : Outport  Port=20
  Cl_Ao : Outport  Port=21
  Ari_Co : Outport  Port=22
  Ali_Bo : Outport  Port=23
  Bo yk : Outport  Port=24
  Brs yk : Outport  Port=25
  wires:
  11 (top) and 12 (bottom)/2 -> <Brs Ao>/1
  11 (top) and 12 (bottom)/3 -> Brs yk/1
  3/2 -> Ali yk/1
  3/1 -> <Ali Bo>/1
  Ari x0/1 -> [Ari], 4/1
  <Cs Bo>/2 -> 9 (top) and 10 (bottom)/1
  <Cs Bo>/8 -> 8/4
  <Cl Ao>/8 -> 7/4
  Co x/1 -> " 5 (bottom) and 6 (top)"/3
  " 5 (bottom) and 6 (top)"/1 -> Co yk/1
  " 5 (bottom) and 6 (top)"/3 -> <Ari Co>/2
  <Ari Co>/8 -> 4/4
  <Ali Bo>/8 -> 3/4
  Ao x/1 -> 1 and 2/3
  Brs x0/1 -> 11 (top) and 12 (bottom)/1, [Brs]
  <Cl Ao>/7 -> [Cl_Ao], 7/3
  <Cl Ao>/2 -> 1 and 2/2
  9 (top) and 10 (bottom)/2 -> <Cs Bo>/2
  <Ari Co>/2 -> " 5 (bottom) and 6 (top)"/2
  7/1 -> <Cl Ao>/1
  Cl x0/1 -> [Cl], 7/1
  4/1 -> <Ari Co>/1
  <Ari Co>/7 -> 4/3, [Ari_Co]
  <Brs Ao>/2 -> 1 and 2/1
  Ao Kz/1 -> 1 and 2/4
  <Brs Ao>/7 -> [Brs_Ao], 11 (top) and 12 (bottom)/6
  <Brs Ao>/8 -> 11 (top) and 12 (bottom)/7
  Co Kz/1 -> " 5 (bottom) and 6 (top)"/4
  8/2 -> Cs yk/1
  Bo Kz/1 -> 9 (top) and 10 (bottom)/4
  1 and 2/3 -> <Cl Ao>/2
  <Brs Co>/8 -> 11 (top) and 12 (bottom)/5
  [Brs12] -> 11 (top) and 12 (bottom)/3
  9 (top) and 10 (bottom)/3 -> <Ali Bo>/2
  <Ali Bo>/7 -> 3/3, [Ali_Bo]
  1 and 2/2 -> <Brs Ao>/2
  Ali x0/1 -> [Ali], 3/1
  <Brs Co>/7 -> 11 (top) and 12 (bottom)/4, [Brs_Co]
  1 and 2/1 -> Ao yk/1
  <Ali Bo>/2 -> 9 (top) and 10 (bottom)/2
  [Ari4] -> 4/2
  8/1 -> <Cs Bo>/1
  4/2 -> Ari yk/1
  <Cs Bo>/7 -> 8/3, [Cs_Bo]
  Cs x0/1 -> [Cs], 8/1
  [Ali3] -> 3/2
  [Brs11] -> 11 (top) and 12 (bottom)/2
  11 (top) and 12 (bottom)/1 -> <Brs Co>/1
  Bo x/1 -> 9 (top) and 10 (bottom)/3
  [Cl7] -> 7/2
  9 (top) and 10 (bottom)/1 -> Bo yk/1
  7/2 -> Cl yk/1
  [Cs8] -> 8/2
  [Ari] -> Ali_Bo/1
  [Ari_Co] -> Ari_Co/1
  [Cl_Ao] -> Cl_Ao/1
  [Cs_Bo] -> Cs_Bo/1
  [Brs_Co] -> Brs_Co/1
  [Brs_Ao] -> Brs_Ao/1
  [Ali] -> Ali/1
  [Ari] -> Ari/1
  [Cl] -> Cl/1
  [Cs] -> Cs/1
  [Brs] -> Brs/1
  Ali3/1 -> [Ali3]
  Ari4/1 -> [Ari4]
  Cl7/1 -> [Cl7]
  Cs8/1 -> [Cs8]
  Brs11/1 -> [Brs11]
  Brs12/1 -> [Brs12]
  1 and 2/4 -> [free_brs12]
  1 and 2/5 -> [free_cl7]
  9 (top) and 10 (bottom)/4 -> [free_cs8]
  9 (top) and 10 (bottom)/5 -> [free_ali3]
  " 5 (bottom) and 6 (top)"/5 -> [free_ari4]
  " 5 (bottom) and 6 (top)"/4 -> [free_brs11]
  [free_cs8] -> free_1/1
  [free_cl7] -> free_2/1
  [free_ari4] -> free_3/1
  [free_ali3] -> free_4/1
  [free_brs12] -> free_5/1
  [free_brs11] -> free_6/1
  <Brs Co>/2 -> " 5 (bottom) and 6 (top)"/1
  " 5 (bottom) and 6 (top)"/2 -> <Brs Co>/2

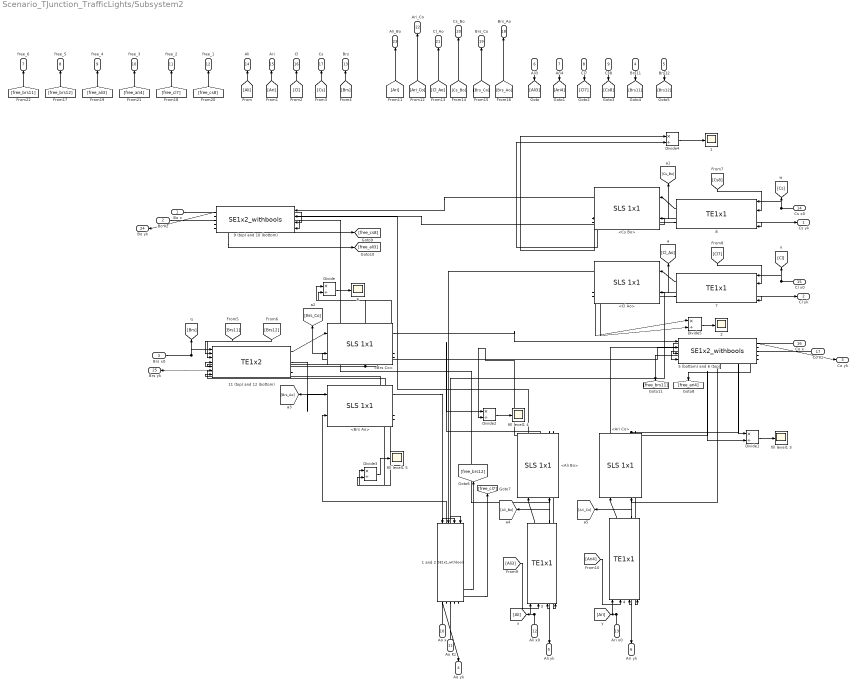
== system Scenario_TJunction_TrafficLights/Subsystem2 ==
  Bo x : Inport
  Bo Kz : Inport  Port=2
  Brs x0 : Inport  Port=3
  Brs11 : Inport  Port=4
  Brs12 : Inport  Port=5
  Ali3 : Inport  Port=6
  Ari4 : Inport  Port=7
  Cl7 : Inport  Port=8
  Cs8 : Inport  Port=9
  Ao x : Inport  Port=10
  Ao Kz : Inport  Port=11
  Ali x0 : Inport  Port=12
  Ari x0 : Inport  Port=13
  Cs x0 : Inport  Port=14
  Cl x0 : Inport  Port=15
  Co x : Inport  Port=16
  Co Kz : Inport  Port=17
  " 5 (bottom) and 6 (top)" : EdgesLibrary/SE1x2_withbools  Rk1=Rk  Rk2=Rk
  1 : Scope
  1 and 2 : EdgesLibrary/SE1x2_withbools  Rk1=Rk  Rk2=Rk
  11 (top) and 12 (bottom) : EdgesLibrary/TE1x2  Rk1=0.5*Rk  Rk2=0.5*Rk
  2 : Scope
  {3..4,7..8} (4 alike) : EdgesLibrary/TE1x1  Rk=Rk
  6 : Scope
  9 (top) and 10 (bottom) : EdgesLibrary/SE1x2_withbools  Rk1=Rk  Rk2=Rk
  <Ali Bo> : StreetLanesLibrary/SLS 1x1  Kz=Kz_left  Tz=Tz_left
  <Ari Co> : StreetLanesLibrary/SLS 1x1  Kz=Kz_right  Tz=Tz_right
  <Brs Ao> : StreetLanesLibrary/SLS 1x1  Kz=Kz_right  Tz=Tz_right
  <Brs Co> : StreetLanesLibrary/SLS 1x1  Kz=Kz_straight  Tz=Tz_straight
  <Cl Ao> : StreetLanesLibrary/SLS 1x1  Kz=Kz_left  Tz=Tz_left
  <Cs Bo> : StreetLanesLibrary/SLS 1x1  Kz=Kz_straight  Tz=Tz_straight
  Divide{,1..5} (6 alike) : Product  Inputs=*/
  fill level1 3 : Scope
  fill level1 4 : Scope
  fill level1 5 : Scope
  Cs yk : Outport
  Cl yk : Outport  Port=2
  Co yk : Outport  Port=3
  Ao yk : Outport  Port=4
  Ali yk : Outport  Port=5
  Ari yk : Outport  Port=6
  free_6 : Outport  Port=7
  free_5 : Outport  Port=8
  free_4 : Outport  Port=9
  free_3 : Outport  Port=10
  free_2 : Outport  Port=11
  free_1 : Outport  Port=12
  Brs : Outport  Port=13
  Ali : Outport  Port=14
  Ari : Outport  Port=15
  Cl : Outport  Port=16
  Cs : Outport  Port=17
  Brs_Ao : Outport  Port=18
  Brs_Co : Outport  Port=19
  Cs_Bo : Outport  Port=20
  Cl_Ao : Outport  Port=21
  Ari_Co : Outport  Port=22
  Ali_Bo : Outport  Port=23
  Bo yk : Outport  Port=24
  Brs yk : Outport  Port=25
  wires:
  11 (top) and 12 (bottom)/2 -> <Brs Ao>/1
  11 (top) and 12 (bottom)/3 -> Brs yk/1
  3/2 -> Ali yk/1
  3/1 -> <Ali Bo>/1
  Ari x0/1 -> [Ari], 4/1
  <Cs Bo>/2 -> 9 (top) and 10 (bottom)/1
  <Cs Bo>/8 -> Divide4/2, 8/4
  <Cl Ao>/8 -> Divide5/2, 7/4
  Co x/1 -> " 5 (bottom) and 6 (top)"/3
  " 5 (bottom) and 6 (top)"/1 -> Co yk/1
  " 5 (bottom) and 6 (top)"/3 -> <Ari Co>/2
  Ao x/1 -> 1 and 2/3
  Brs x0/1 -> 11 (top) and 12 (bottom)/1, [Brs]
  <Cl Ao>/7 -> Divide5/1, [Cl_Ao], 7/3
  <Cl Ao>/2 -> 1 and 2/2
  9 (top) and 10 (bottom)/2 -> <Cs Bo>/2
  <Ari Co>/2 -> " 5 (bottom) and 6 (top)"/2
  7/1 -> <Cl Ao>/1
  Cl x0/1 -> [Cl], 7/1
  4/1 -> <Ari Co>/1
  <Brs Ao>/2 -> 1 and 2/1
  Ao Kz/1 -> 1 and 2/4
  Co Kz/1 -> " 5 (bottom) and 6 (top)"/4
  8/2 -> Cs yk/1
  Bo Kz/1 -> 9 (top) and 10 (bottom)/4
  1 and 2/3 -> <Cl Ao>/2
  <Brs Co>/8 -> Divide/2, 11 (top) and 12 (bottom)/5
  [Brs12] -> 11 (top) and 12 (bottom)/3
  9 (top) and 10 (bottom)/3 -> <Ali Bo>/2
  1 and 2/2 -> <Brs Ao>/2
  Ali x0/1 -> [Ali], 3/1
  <Brs Co>/7 -> Divide/1, 11 (top) and 12 (bottom)/4, [Brs_Co]
  1 and 2/1 -> Ao yk/1
  <Ali Bo>/2 -> 9 (top) and 10 (bottom)/2
  [Ari4] -> 4/2
  8/1 -> <Cs Bo>/1
  4/2 -> Ari yk/1
  <Cs Bo>/7 -> Divide4/1, 8/3, [Cs_Bo]
  Cs x0/1 -> [Cs], 8/1
  [Ali3] -> 3/2
  [Brs11] -> 11 (top) and 12 (bottom)/2
  11 (top) and 12 (bottom)/1 -> <Brs Co>/1
  Bo x/1 -> 9 (top) and 10 (bottom)/3
  [Cl7] -> 7/2
  9 (top) and 10 (bottom)/1 -> Bo yk/1
  7/2 -> Cl yk/1
  [Cs8] -> 8/2
  [Ari] -> Ali_Bo/1
  [Ari_Co] -> Ari_Co/1
  [Cl_Ao] -> Cl_Ao/1
  [Cs_Bo] -> Cs_Bo/1
  [Brs_Co] -> Brs_Co/1
  [Brs_Ao] -> Brs_Ao/1
  [Ali] -> Ali/1
  [Ari] -> Ari/1
  [Cl] -> Cl/1
  [Cs] -> Cs/1
  [Brs] -> Brs/1
  Ali3/1 -> [Ali3]
  Ari4/1 -> [Ari4]
  Cl7/1 -> [Cl7]
  Cs8/1 -> [Cs8]
  Brs11/1 -> [Brs11]
  Brs12/1 -> [Brs12]
  1 and 2/4 -> [free_brs12]
  1 and 2/5 -> [free_cl7]
  9 (top) and 10 (bottom)/4 -> [free_cs8]
  9 (top) and 10 (bottom)/5 -> [free_ali3]
  " 5 (bottom) and 6 (top)"/5 -> [free_ari4]
  " 5 (bottom) and 6 (top)"/4 -> [free_brs11]
  [free_cs8] -> free_1/1
  [free_cl7] -> free_2/1
  [free_ari4] -> free_3/1
  [free_ali3] -> free_4/1
  [free_brs12] -> free_5/1
  [free_brs11] -> free_6/1
  <Brs Co>/2 -> " 5 (bottom) and 6 (top)"/1
  " 5 (bottom) and 6 (top)"/2 -> <Brs Co>/2
  <Ari Co>/8 -> Divide1/2, 4/4
  <Ari Co>/7 -> 4/3, [Ari_Co], Divide1/1
  Divide1/1 -> fill level1 3/1
  Divide2/1 -> fill level1 4/1
  <Ali Bo>/7 -> Divide2/1, 3/3, [Ali_Bo]
  <Ali Bo>/8 -> Divide2/2, 3/4
  Divide3/1 -> fill level1 5/1
  <Brs Ao>/7 -> [Brs_Ao], 11 (top) and 12 (bottom)/6, Divide3/1
  <Brs Ao>/8 -> Divide3/2, 11 (top) and 12 (bottom)/7
  Divide/1 -> 6/1
  Divide4/1 -> 1/1
  Divide5/1 -> 2/1
